simulink subsystem "AFO_Hopf_network"  (R2020a)
settings: Solver=VariableStepAuto  StartTime=0.0  StopTime=10.0  RelTol=1e-3
PreLoadFcn:
  | addpath(pwd);
settings Model: Creator=12927  LastModifiedBy=12927

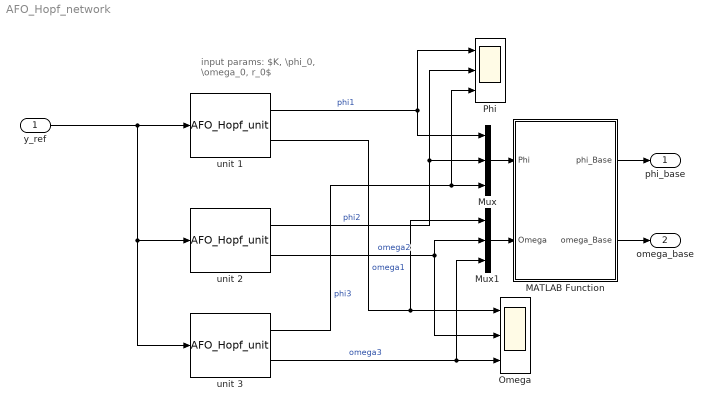
== system AFO_Hopf_network ==
  note: input params:
      | $K, \phi_0, \omega_0, r_0$
  y_ref : Inport
  MATLAB Function : MATLAB Function  TreatAsAtomicUnit=on
  Mux : Mux  Inputs=3
  Mux1 : Mux  Inputs=3
  Omega : Scope  NumInputPorts=3
  Phi : Scope  NumInputPorts=3
  unit 1 : M-S-Function  FunctionName=AFO_Hopf_unit  Parameters=10,0,0.5,1
  unit 2 : M-S-Function  FunctionName=AFO_Hopf_unit  Parameters=10,0,1,1
  unit 3 : M-S-Function  FunctionName=AFO_Hopf_unit  Parameters=10,0,2,1
  phi_base : Outport
  omega_base : Outport  Port=2
  wires:
  unit 1/1 -> Mux/1, Phi/1  "phi1"
  y_ref/1 -> unit 1/1, unit 2/1, unit 3/1
  unit 1/2 -> Omega/1, Mux1/1  "omega1"
  Mux/1 -> MATLAB Function/1(Phi)
  Mux1/1 -> MATLAB Function/2(Omega)
  MATLAB Function/2(omega_Base) -> omega_base/1
  MATLAB Function/1(phi_Base) -> phi_base/1
  unit 2/1 -> Phi/2, Mux/2  "phi2"
  unit 2/2 -> Mux1/2, Omega/2  "omega2"
  unit 3/1 -> Mux/3, Phi/3  "phi3"
  unit 3/2 -> Mux1/3, Omega/3  "omega3"

== matlab function AFO_Hopf_network/MATLAB Function ==
  data: Phi input; phi_Base output; Omega input; omega_Base output
function [phi_Base, omega_Base] = selectBaseSignal(Phi, Omega)

index1 = find(Omega);
Phi = Phi(index1);
[omega_Base, indexMin] = min(Omega(index1)); 
phi_Base = Phi(indexMin);
